simulink model "VCU_CS75_12_16_Test"  (R2014a)
settings: Solver=FixedStepDiscrete  StartTime=0.0  StopTime=25  FixedStep=0.0005  RelTol=1e-3
undefined symbols (not defined in the file): ecucoder_acal, I_SW01_L, LaterlAngleCommand, LDW, RemoteAcclPosition
libraries: simulink x913, ec5744lib x39
(part 17 of 30)

== system VCU_CS75_12_16_Test/长安CS75底盘程序，20ms一次/Output/Subsystem/28A/APA_28A/APA_IncreasePressureReq ==
  APA_IncreasePressureReq : Inport
  APA_IncreasePressureReqRon : Rounding  Operator=round
  APA_IncreasePressureReq_1sat : Saturate  UpperLimit=128  LowerLimit=0
  APA_IncreasePressureReq_Convert : DataTypeConversion  OutDataTypeStr=uint8
  APA_IncreasePressureReq_Convert1 : DataTypeConversion  OutDataTypeStr=uint32
  APA_IncreasePressureReq_D : Product  Inputs=*/
  APA_IncreasePressureReq_F : Constant  OutDataTypeStr=single
  APA_IncreasePressureReq_L : simulink/Logic and Bit Operations/Bitwise Operator  logicop=AND  UseBitMask=on  BitMask=128  BitMaskRealWorld=Stored Integer
  APA_IncreasePressureReq_O : Constant  Value=0  OutDataTypeStr=single
  APA_IncreasePressureReq_S : ArithShift  BitShiftNumber=-7
  APA_IncreasePressureReq_sat : Saturate  UpperLimit=0  LowerLimit=0
  APA_IncreasePressureReq_st : Sum  Inputs=+-
  Constant{1,3..8} (7 alike) : Constant  Value=0  OutDataTypeStr=uint8
  output1 : Outport
  output2 : Outport  Port=2
  output3 : Outport  Port=3
  output4 : Outport  Port=4
  output5 : Outport  Port=5
  output6 : Outport  Port=6
  output7 : Outport  Port=7
  output8 : Outport  Port=8
  wires:
  Constant8/1 -> output8/1
  Constant7/1 -> output7/1
  Constant6/1 -> output6/1
  Constant5/1 -> output5/1
  Constant4/1 -> output4/1
  Constant3/1 -> output3/1
  Constant1/1 -> output1/1
  APA_IncreasePressureReq_Convert/1 -> output2/1
  APA_IncreasePressureReq_L/1 -> APA_IncreasePressureReq_Convert/1
  APA_IncreasePressureReq_Convert1/1 -> APA_IncreasePressureReq_L/1
  APA_IncreasePressureReq_1sat/1 -> APA_IncreasePressureReq_Convert1/1
  APA_IncreasePressureReq_S/1 -> APA_IncreasePressureReq_1sat/1
  APA_IncreasePressureReqRon/1 -> APA_IncreasePressureReq_S/1
  APA_IncreasePressureReq_D/1 -> APA_IncreasePressureReqRon/1
  APA_IncreasePressureReq_F/1 -> APA_IncreasePressureReq_D/2
  APA_IncreasePressureReq_st/1 -> APA_IncreasePressureReq_D/1
  APA_IncreasePressureReq_O/1 -> APA_IncreasePressureReq_st/2
  APA_IncreasePressureReq_sat/1 -> APA_IncreasePressureReq_st/1
  APA_IncreasePressureReq/1 -> APA_IncreasePressureReq_sat/1

== system VCU_CS75_12_16_Test/长安CS75底盘程序，20ms一次/Output/Subsystem/28A/APA_28A/APA_Indication ==
  APA_Indication : Inport
  APA_IndicationRon : Rounding  Operator=round
  APA_Indication_1sat : Saturate  UpperLimit=56  LowerLimit=0
  APA_Indication_Convert : DataTypeConversion  OutDataTypeStr=uint8
  APA_Indication_Convert1 : DataTypeConversion  OutDataTypeStr=uint32
  APA_Indication_D : Product  Inputs=*/
  APA_Indication_F : Constant  OutDataTypeStr=single
  APA_Indication_L : simulink/Logic and Bit Operations/Bitwise Operator  logicop=AND  UseBitMask=on  BitMask=56  BitMaskRealWorld=Stored Integer
  APA_Indication_O : Constant  Value=0  OutDataTypeStr=single
  APA_Indication_S : ArithShift  BitShiftNumber=-3
  APA_Indication_sat : Saturate  UpperLimit=7  LowerLimit=0
  APA_Indication_st : Sum  Inputs=+-
  Constant{2..8} (7 alike) : Constant  Value=0  OutDataTypeStr=uint8
  output1 : Outport
  output2 : Outport  Port=2
  output3 : Outport  Port=3
  output4 : Outport  Port=4
  output5 : Outport  Port=5
  output6 : Outport  Port=6
  output7 : Outport  Port=7
  output8 : Outport  Port=8
  wires:
  Constant8/1 -> output8/1
  Constant7/1 -> output7/1
  Constant6/1 -> output6/1
  Constant5/1 -> output5/1
  Constant4/1 -> output4/1
  Constant3/1 -> output3/1
  Constant2/1 -> output2/1
  APA_Indication_Convert/1 -> output1/1
  APA_Indication_L/1 -> APA_Indication_Convert/1
  APA_Indication_Convert1/1 -> APA_Indication_L/1
  APA_Indication_1sat/1 -> APA_Indication_Convert1/1
  APA_Indication_S/1 -> APA_Indication_1sat/1
  APA_IndicationRon/1 -> APA_Indication_S/1
  APA_Indication_D/1 -> APA_IndicationRon/1
  APA_Indication_F/1 -> APA_Indication_D/2
  APA_Indication_st/1 -> APA_Indication_D/1
  APA_Indication_O/1 -> APA_Indication_st/2
  APA_Indication_sat/1 -> APA_Indication_st/1
  APA_Indication/1 -> APA_Indication_sat/1

== system VCU_CS75_12_16_Test/长安CS75底盘程序，20ms一次/Output/Subsystem/28A/APA_28A/APA_OnOff ==
  APA_OnOff : Inport
  APA_OnOffRon : Rounding  Operator=round
  APA_OnOff_1sat : Saturate  UpperLimit=64  LowerLimit=0
  APA_OnOff_Convert : DataTypeConversion  OutDataTypeStr=uint8
  APA_OnOff_Convert1 : DataTypeConversion  OutDataTypeStr=uint32
  APA_OnOff_D : Product  Inputs=*/
  APA_OnOff_F : Constant  OutDataTypeStr=single
  APA_OnOff_L : simulink/Logic and Bit Operations/Bitwise Operator  logicop=AND  UseBitMask=on  BitMask=64  BitMaskRealWorld=Stored Integer
  APA_OnOff_O : Constant  Value=0  OutDataTypeStr=single
  APA_OnOff_S : ArithShift  BitShiftNumber=-6
  APA_OnOff_sat : Saturate  UpperLimit=0  LowerLimit=0
  APA_OnOff_st : Sum  Inputs=+-
  Constant{2..8} (7 alike) : Constant  Value=0  OutDataTypeStr=uint8
  output1 : Outport
  output2 : Outport  Port=2
  output3 : Outport  Port=3
  output4 : Outport  Port=4
  output5 : Outport  Port=5
  output6 : Outport  Port=6
  output7 : Outport  Port=7
  output8 : Outport  Port=8
  wires:
  Constant8/1 -> output8/1
  Constant7/1 -> output7/1
  Constant6/1 -> output6/1
  Constant5/1 -> output5/1
  Constant4/1 -> output4/1
  Constant3/1 -> output3/1
  Constant2/1 -> output2/1
  APA_OnOff_Convert/1 -> output1/1
  APA_OnOff_L/1 -> APA_OnOff_Convert/1
  APA_OnOff_Convert1/1 -> APA_OnOff_L/1
  APA_OnOff_1sat/1 -> APA_OnOff_Convert1/1
  APA_OnOff_S/1 -> APA_OnOff_1sat/1
  APA_OnOffRon/1 -> APA_OnOff_S/1
  APA_OnOff_D/1 -> APA_OnOffRon/1
  APA_OnOff_F/1 -> APA_OnOff_D/2
  APA_OnOff_st/1 -> APA_OnOff_D/1
  APA_OnOff_O/1 -> APA_OnOff_st/2
  APA_OnOff_sat/1 -> APA_OnOff_st/1
  APA_OnOff/1 -> APA_OnOff_sat/1

== system VCU_CS75_12_16_Test/长安CS75底盘程序，20ms一次/Output/Subsystem/28A/APA_28A/APA_RollingCounter ==
  APA_RollingCounter : Inport
  APA_RollingCounterRon : Rounding  Operator=round
  APA_RollingCounter_1sat : Saturate  UpperLimit=15  LowerLimit=0
  APA_RollingCounter_Convert : DataTypeConversion  OutDataTypeStr=uint8
  APA_RollingCounter_Convert1 : DataTypeConversion  OutDataTypeStr=uint32
  APA_RollingCounter_D : Product  Inputs=*/
  APA_RollingCounter_F : Constant  OutDataTypeStr=single
  APA_RollingCounter_L : simulink/Logic and Bit Operations/Bitwise Operator  logicop=AND  UseBitMask=on  BitMask=15  BitMaskRealWorld=Stored Integer
  APA_RollingCounter_O : Constant  Value=0  OutDataTypeStr=single
  APA_RollingCounter_S : ArithShift
  APA_RollingCounter_sat : Saturate  UpperLimit=15  LowerLimit=0
  APA_RollingCounter_st : Sum  Inputs=+-
  Constant{1..6,8} (7 alike) : Constant  Value=0  OutDataTypeStr=uint8
  output1 : Outport
  output2 : Outport  Port=2
  output3 : Outport  Port=3
  output4 : Outport  Port=4
  output5 : Outport  Port=5
  output6 : Outport  Port=6
  output7 : Outport  Port=7
  output8 : Outport  Port=8
  wires:
  Constant8/1 -> output8/1
  Constant6/1 -> output6/1
  Constant5/1 -> output5/1
  Constant4/1 -> output4/1
  Constant3/1 -> output3/1
  Constant2/1 -> output2/1
  Constant1/1 -> output1/1
  APA_RollingCounter_Convert/1 -> output7/1
  APA_RollingCounter_L/1 -> APA_RollingCounter_Convert/1
  APA_RollingCounter_Convert1/1 -> APA_RollingCounter_L/1
  APA_RollingCounter_1sat/1 -> APA_RollingCounter_Convert1/1
  APA_RollingCounter_S/1 -> APA_RollingCounter_1sat/1
  APA_RollingCounterRon/1 -> APA_RollingCounter_S/1
  APA_RollingCounter_D/1 -> APA_RollingCounterRon/1
  APA_RollingCounter_F/1 -> APA_RollingCounter_D/2
  APA_RollingCounter_st/1 -> APA_RollingCounter_D/1
  APA_RollingCounter_O/1 -> APA_RollingCounter_st/2
  APA_RollingCounter_sat/1 -> APA_RollingCounter_st/1
  APA_RollingCounter/1 -> APA_RollingCounter_sat/1

== system VCU_CS75_12_16_Test/长安CS75底盘程序，20ms一次/Output/Subsystem/28A/APA_28A/APA_SteeringAngleReqProtection ==
  APA_SteeringAngleReqProtection : Inport
  APA_SteeringAngleReqProtectionRon : Rounding  Operator=round
  APA_SteeringAngleReqProtection_1sat : Saturate  UpperLimit=3  LowerLimit=0
  APA_SteeringAngleReqProtection_Convert : DataTypeConversion  OutDataTypeStr=uint8
  APA_SteeringAngleReqProtection_Convert1 : DataTypeConversion  OutDataTypeStr=uint32
  APA_SteeringAngleReqProtection_D : Product  Inputs=*/
  APA_SteeringAngleReqProtection_F : Constant  OutDataTypeStr=single
  APA_SteeringAngleReqProtection_L : simulink/Logic and Bit Operations/Bitwise Operator  logicop=AND  UseBitMask=on  BitMask=3  BitMaskRealWorld=Stored Integer
  APA_SteeringAngleReqProtection_O : Constant  Value=0  OutDataTypeStr=single
  APA_SteeringAngleReqProtection_S : ArithShift
  APA_SteeringAngleReqProtection_sat : Saturate  UpperLimit=3  LowerLimit=0
  APA_SteeringAngleReqProtection_st : Sum  Inputs=+-
  Constant{1..4,6..8} (7 alike) : Constant  Value=0  OutDataTypeStr=uint8
  output1 : Outport
  output2 : Outport  Port=2
  output3 : Outport  Port=3
  output4 : Outport  Port=4
  output5 : Outport  Port=5
  output6 : Outport  Port=6
  output7 : Outport  Port=7
  output8 : Outport  Port=8
  wires:
  Constant8/1 -> output8/1
  Constant7/1 -> output7/1
  Constant6/1 -> output6/1
  Constant4/1 -> output4/1
  Constant3/1 -> output3/1
  Constant2/1 -> output2/1
  Constant1/1 -> output1/1
  APA_SteeringAngleReqProtection_Convert/1 -> output5/1
  APA_SteeringAngleReqProtection_L/1 -> APA_SteeringAngleReqProtection_Convert/1
  APA_SteeringAngleReqProtection_Convert1/1 -> APA_SteeringAngleReqProtection_L/1
  APA_SteeringAngleReqProtection_1sat/1 -> APA_SteeringAngleReqProtection_Convert1/1
  APA_SteeringAngleReqProtection_S/1 -> APA_SteeringAngleReqProtection_1sat/1
  APA_SteeringAngleReqProtectionRon/1 -> APA_SteeringAngleReqProtection_S/1
  APA_SteeringAngleReqProtection_D/1 -> APA_SteeringAngleReqProtectionRon/1
  APA_SteeringAngleReqProtection_F/1 -> APA_SteeringAngleReqProtection_D/2
  APA_SteeringAngleReqProtection_st/1 -> APA_SteeringAngleReqProtection_D/1
  APA_SteeringAngleReqProtection_O/1 -> APA_SteeringAngleReqProtection_st/2
  APA_SteeringAngleReqProtection_sat/1 -> APA_SteeringAngleReqProtection_st/1
  APA_SteeringAngleReqProtection/1 -> APA_SteeringAngleReqProtection_sat/1

== system VCU_CS75_12_16_Test/长安CS75底盘程序，20ms一次/Output/Subsystem/28D/LAS_28D/CRC ==
  CRC : Inport
  CRCRon : Rounding  Operator=round
  CRC_1sat : Saturate  UpperLimit=255  LowerLimit=0
  CRC_Convert : DataTypeConversion  OutDataTypeStr=uint8
  CRC_Convert1 : DataTypeConversion  OutDataTypeStr=uint32
  CRC_D : Product  Inputs=*/
  CRC_F : Constant  OutDataTypeStr=single
  CRC_L : simulink/Logic and Bit Operations/Bitwise Operator  logicop=AND  UseBitMask=on  BitMask=255  BitMaskRealWorld=Stored Integer
  CRC_O : Constant  Value=0  OutDataTypeStr=single
  CRC_S : ArithShift
  CRC_sat : Saturate  UpperLimit=0  LowerLimit=0
  CRC_st : Sum  Inputs=+-
  Constant{1..7} (7 alike) : Constant  Value=0  OutDataTypeStr=uint8
  output1 : Outport
  output2 : Outport  Port=2
  output3 : Outport  Port=3
  output4 : Outport  Port=4
  output5 : Outport  Port=5
  output6 : Outport  Port=6
  output7 : Outport  Port=7
  output8 : Outport  Port=8
  wires:
  CRC/1 -> CRC_sat/1
  CRC_sat/1 -> CRC_st/1
  CRC_O/1 -> CRC_st/2
  CRC_st/1 -> CRC_D/1
  CRC_F/1 -> CRC_D/2
  CRC_D/1 -> CRCRon/1
  CRCRon/1 -> CRC_S/1
  CRC_S/1 -> CRC_1sat/1
  CRC_1sat/1 -> CRC_Convert1/1
  CRC_Convert1/1 -> CRC_L/1
  CRC_L/1 -> CRC_Convert/1
  CRC_Convert/1 -> output8/1
  Constant1/1 -> output1/1
  Constant2/1 -> output2/1
  Constant3/1 -> output3/1
  Constant4/1 -> output4/1
  Constant5/1 -> output5/1
  Constant6/1 -> output6/1
  Constant7/1 -> output7/1

== system VCU_CS75_12_16_Test/长安CS75底盘程序，20ms一次/Output/Subsystem/28D/LAS_28D/LAS_CaliStatus ==
  LAS_CaliStatus : Inport
  Constant{1,3..8} (7 alike) : Constant  Value=0  OutDataTypeStr=uint8
  LAS_CaliStatusRon : Rounding  Operator=round
  LAS_CaliStatus_1sat : Saturate  UpperLimit=3  LowerLimit=0
  LAS_CaliStatus_Convert : DataTypeConversion  OutDataTypeStr=uint8
  LAS_CaliStatus_Convert1 : DataTypeConversion  OutDataTypeStr=uint32
  LAS_CaliStatus_D : Product  Inputs=*/
  LAS_CaliStatus_F : Constant  OutDataTypeStr=single
  LAS_CaliStatus_L : simulink/Logic and Bit Operations/Bitwise Operator  logicop=AND  UseBitMask=on  BitMask=3  BitMaskRealWorld=Stored Integer
  LAS_CaliStatus_O : Constant  Value=0  OutDataTypeStr=single
  LAS_CaliStatus_S : ArithShift
  LAS_CaliStatus_sat : Saturate  UpperLimit=0  LowerLimit=0
  LAS_CaliStatus_st : Sum  Inputs=+-
  output1 : Outport
  output2 : Outport  Port=2
  output3 : Outport  Port=3
  output4 : Outport  Port=4
  output5 : Outport  Port=5
  output6 : Outport  Port=6
  output7 : Outport  Port=7
  output8 : Outport  Port=8
  wires:
  LAS_CaliStatus/1 -> LAS_CaliStatus_sat/1
  LAS_CaliStatus_sat/1 -> LAS_CaliStatus_st/1
  LAS_CaliStatus_O/1 -> LAS_CaliStatus_st/2
  LAS_CaliStatus_st/1 -> LAS_CaliStatus_D/1
  LAS_CaliStatus_F/1 -> LAS_CaliStatus_D/2
  LAS_CaliStatus_D/1 -> LAS_CaliStatusRon/1
  LAS_CaliStatusRon/1 -> LAS_CaliStatus_S/1
  LAS_CaliStatus_S/1 -> LAS_CaliStatus_1sat/1
  LAS_CaliStatus_1sat/1 -> LAS_CaliStatus_Convert1/1
  LAS_CaliStatus_Convert1/1 -> LAS_CaliStatus_L/1
  LAS_CaliStatus_L/1 -> LAS_CaliStatus_Convert/1
  LAS_CaliStatus_Convert/1 -> output2/1
  Constant1/1 -> output1/1
  Constant3/1 -> output3/1
  Constant4/1 -> output4/1
  Constant5/1 -> output5/1
  Constant6/1 -> output6/1
  Constant7/1 -> output7/1
  Constant8/1 -> output8/1

== system VCU_CS75_12_16_Test/长安CS75底盘程序，20ms一次/Output/Subsystem/28D/LAS_28D/LAS_DFDFailed ==
  LAS_DFDFailed : Inport
  Constant{1,3..8} (7 alike) : Constant  Value=0  OutDataTypeStr=uint8
  LAS_DFDFailedRon : Rounding  Operator=round
  LAS_DFDFailed_1sat : Saturate  UpperLimit=8  LowerLimit=0
  LAS_DFDFailed_Convert : DataTypeConversion  OutDataTypeStr=uint8
  LAS_DFDFailed_Convert1 : DataTypeConversion  OutDataTypeStr=uint32
  LAS_DFDFailed_D : Product  Inputs=*/
  LAS_DFDFailed_F : Constant  OutDataTypeStr=single
  LAS_DFDFailed_L : simulink/Logic and Bit Operations/Bitwise Operator  logicop=AND  UseBitMask=on  BitMask=8  BitMaskRealWorld=Stored Integer
  LAS_DFDFailed_O : Constant  Value=0  OutDataTypeStr=single
  LAS_DFDFailed_S : ArithShift  BitShiftNumber=-3
  LAS_DFDFailed_sat : Saturate  UpperLimit=0  LowerLimit=0
  LAS_DFDFailed_st : Sum  Inputs=+-
  output1 : Outport
  output2 : Outport  Port=2
  output3 : Outport  Port=3
  output4 : Outport  Port=4
  output5 : Outport  Port=5
  output6 : Outport  Port=6
  output7 : Outport  Port=7
  output8 : Outport  Port=8
  wires:
  LAS_DFDFailed/1 -> LAS_DFDFailed_sat/1
  LAS_DFDFailed_sat/1 -> LAS_DFDFailed_st/1
  LAS_DFDFailed_O/1 -> LAS_DFDFailed_st/2
  LAS_DFDFailed_st/1 -> LAS_DFDFailed_D/1
  LAS_DFDFailed_F/1 -> LAS_DFDFailed_D/2
  LAS_DFDFailed_D/1 -> LAS_DFDFailedRon/1
  LAS_DFDFailedRon/1 -> LAS_DFDFailed_S/1
  LAS_DFDFailed_S/1 -> LAS_DFDFailed_1sat/1
  LAS_DFDFailed_1sat/1 -> LAS_DFDFailed_Convert1/1
  LAS_DFDFailed_Convert1/1 -> LAS_DFDFailed_L/1
  LAS_DFDFailed_L/1 -> LAS_DFDFailed_Convert/1
  LAS_DFDFailed_Convert/1 -> output2/1
  Constant1/1 -> output1/1
  Constant3/1 -> output3/1
  Constant4/1 -> output4/1
  Constant5/1 -> output5/1
  Constant6/1 -> output6/1
  Constant7/1 -> output7/1
  Constant8/1 -> output8/1

== system VCU_CS75_12_16_Test/长安CS75底盘程序，20ms一次/Output/Subsystem/28D/LAS_28D/LAS_DFDWarning ==
  LAS_DFDWarning : Inport
  Constant{1..3,5..8} (7 alike) : Constant  Value=0  OutDataTypeStr=uint8
  LAS_DFDWarningRon : Rounding  Operator=round
  LAS_DFDWarning_1sat : Saturate  UpperLimit=3  LowerLimit=0
  LAS_DFDWarning_Convert : DataTypeConversion  OutDataTypeStr=uint8
  LAS_DFDWarning_Convert1 : DataTypeConversion  OutDataTypeStr=uint32
  LAS_DFDWarning_D : Product  Inputs=*/
  LAS_DFDWarning_F : Constant  OutDataTypeStr=single
  LAS_DFDWarning_L : simulink/Logic and Bit Operations/Bitwise Operator  logicop=AND  UseBitMask=on  BitMask=3  BitMaskRealWorld=Stored Integer
  LAS_DFDWarning_O : Constant  Value=0  OutDataTypeStr=single
  LAS_DFDWarning_S : ArithShift
  LAS_DFDWarning_sat : Saturate  UpperLimit=0  LowerLimit=0
  LAS_DFDWarning_st : Sum  Inputs=+-
  output1 : Outport
  output2 : Outport  Port=2
  output3 : Outport  Port=3
  output4 : Outport  Port=4
  output5 : Outport  Port=5
  output6 : Outport  Port=6
  output7 : Outport  Port=7
  output8 : Outport  Port=8
  wires:
  LAS_DFDWarning/1 -> LAS_DFDWarning_sat/1
  LAS_DFDWarning_sat/1 -> LAS_DFDWarning_st/1
  LAS_DFDWarning_O/1 -> LAS_DFDWarning_st/2
  LAS_DFDWarning_st/1 -> LAS_DFDWarning_D/1
  LAS_DFDWarning_F/1 -> LAS_DFDWarning_D/2
  LAS_DFDWarning_D/1 -> LAS_DFDWarningRon/1
  LAS_DFDWarningRon/1 -> LAS_DFDWarning_S/1
  LAS_DFDWarning_S/1 -> LAS_DFDWarning_1sat/1
  LAS_DFDWarning_1sat/1 -> LAS_DFDWarning_Convert1/1
  LAS_DFDWarning_Convert1/1 -> LAS_DFDWarning_L/1
  LAS_DFDWarning_L/1 -> LAS_DFDWarning_Convert/1
  LAS_DFDWarning_Convert/1 -> output4/1
  Constant1/1 -> output1/1
  Constant2/1 -> output2/1
  Constant3/1 -> output3/1
  Constant5/1 -> output5/1
  Constant6/1 -> output6/1
  Constant7/1 -> output7/1
  Constant8/1 -> output8/1

== system VCU_CS75_12_16_Test/长安CS75底盘程序，20ms一次/Output/Subsystem/28D/LAS_28D/LAS_LASFailed ==
  LAS_LASFailed : Inport
  Constant{1..3,5..8} (7 alike) : Constant  Value=0  OutDataTypeStr=uint8
  LAS_LASFailedRon : Rounding  Operator=round
  LAS_LASFailed_1sat : Saturate  UpperLimit=12  LowerLimit=0
  LAS_LASFailed_Convert : DataTypeConversion  OutDataTypeStr=uint8
  LAS_LASFailed_Convert1 : DataTypeConversion  OutDataTypeStr=uint32
  LAS_LASFailed_D : Product  Inputs=*/
  LAS_LASFailed_F : Constant  OutDataTypeStr=single
  LAS_LASFailed_L : simulink/Logic and Bit Operations/Bitwise Operator  logicop=AND  UseBitMask=on  BitMask=12  BitMaskRealWorld=Stored Integer
  LAS_LASFailed_O : Constant  Value=0  OutDataTypeStr=single
  LAS_LASFailed_S : ArithShift  BitShiftNumber=-2
  LAS_LASFailed_sat : Saturate  UpperLimit=0  LowerLimit=0
  LAS_LASFailed_st : Sum  Inputs=+-
  output1 : Outport
  output2 : Outport  Port=2
  output3 : Outport  Port=3
  output4 : Outport  Port=4
  output5 : Outport  Port=5
  output6 : Outport  Port=6
  output7 : Outport  Port=7
  output8 : Outport  Port=8
  wires:
  LAS_LASFailed/1 -> LAS_LASFailed_sat/1
  LAS_LASFailed_sat/1 -> LAS_LASFailed_st/1
  LAS_LASFailed_O/1 -> LAS_LASFailed_st/2
  LAS_LASFailed_st/1 -> LAS_LASFailed_D/1
  LAS_LASFailed_F/1 -> LAS_LASFailed_D/2
  LAS_LASFailed_D/1 -> LAS_LASFailedRon/1
  LAS_LASFailedRon/1 -> LAS_LASFailed_S/1
  LAS_LASFailed_S/1 -> LAS_LASFailed_1sat/1
  LAS_LASFailed_1sat/1 -> LAS_LASFailed_Convert1/1
  LAS_LASFailed_Convert1/1 -> LAS_LASFailed_L/1
  LAS_LASFailed_L/1 -> LAS_LASFailed_Convert/1
  LAS_LASFailed_Convert/1 -> output4/1
  Constant1/1 -> output1/1
  Constant2/1 -> output2/1
  Constant3/1 -> output3/1
  Constant5/1 -> output5/1
  Constant6/1 -> output6/1
  Constant7/1 -> output7/1
  Constant8/1 -> output8/1

== system VCU_CS75_12_16_Test/长安CS75底盘程序，20ms一次/Output/Subsystem/28D/LAS_28D/LAS_LDWReminder ==
  LAS_LDWReminder : Inport
  Constant{1..2,4..8} (7 alike) : Constant  Value=0  OutDataTypeStr=uint8
  LAS_LDWReminderRon : Rounding  Operator=round
  LAS_LDWReminder_1sat : Saturate  UpperLimit=96  LowerLimit=0
  LAS_LDWReminder_Convert : DataTypeConversion  OutDataTypeStr=uint8
  LAS_LDWReminder_Convert1 : DataTypeConversion  OutDataTypeStr=uint32
  LAS_LDWReminder_D : Product  Inputs=*/
  LAS_LDWReminder_F : Constant  OutDataTypeStr=single
  LAS_LDWReminder_L : simulink/Logic and Bit Operations/Bitwise Operator  logicop=AND  UseBitMask=on  BitMask=96  BitMaskRealWorld=Stored Integer
  LAS_LDWReminder_O : Constant  Value=0  OutDataTypeStr=single
  LAS_LDWReminder_S : ArithShift  BitShiftNumber=-5
  LAS_LDWReminder_sat : Saturate  UpperLimit=0  LowerLimit=0
  LAS_LDWReminder_st : Sum  Inputs=+-
  output1 : Outport
  output2 : Outport  Port=2
  output3 : Outport  Port=3
  output4 : Outport  Port=4
  output5 : Outport  Port=5
  output6 : Outport  Port=6
  output7 : Outport  Port=7
  output8 : Outport  Port=8
  wires:
  LAS_LDWReminder/1 -> LAS_LDWReminder_sat/1
  LAS_LDWReminder_sat/1 -> LAS_LDWReminder_st/1
  LAS_LDWReminder_O/1 -> LAS_LDWReminder_st/2
  LAS_LDWReminder_st/1 -> LAS_LDWReminder_D/1
  LAS_LDWReminder_F/1 -> LAS_LDWReminder_D/2
  LAS_LDWReminder_D/1 -> LAS_LDWReminderRon/1
  LAS_LDWReminderRon/1 -> LAS_LDWReminder_S/1
  LAS_LDWReminder_S/1 -> LAS_LDWReminder_1sat/1
  LAS_LDWReminder_1sat/1 -> LAS_LDWReminder_Convert1/1
  LAS_LDWReminder_Convert1/1 -> LAS_LDWReminder_L/1
  LAS_LDWReminder_L/1 -> LAS_LDWReminder_Convert/1
  LAS_LDWReminder_Convert/1 -> output3/1
  Constant1/1 -> output1/1
  Constant2/1 -> output2/1
  Constant4/1 -> output4/1
  Constant5/1 -> output5/1
  Constant6/1 -> output6/1
  Constant7/1 -> output7/1
  Constant8/1 -> output8/1

== system VCU_CS75_12_16_Test/长安CS75底盘程序，20ms一次/Output/Subsystem/28D/LAS_28D/LAS_LDWStatus ==
  LAS_LDWStatus : Inport
  Constant{2..8} (7 alike) : Constant  Value=0  OutDataTypeStr=uint8
  LAS_LDWStatusRon : Rounding  Operator=round
  LAS_LDWStatus_1sat : Saturate  UpperLimit=96  LowerLimit=0
  LAS_LDWStatus_Convert : DataTypeConversion  OutDataTypeStr=uint8
  LAS_LDWStatus_Convert1 : DataTypeConversion  OutDataTypeStr=uint32
  LAS_LDWStatus_D : Product  Inputs=*/
  LAS_LDWStatus_F : Constant  OutDataTypeStr=single
  LAS_LDWStatus_L : simulink/Logic and Bit Operations/Bitwise Operator  logicop=AND  UseBitMask=on  BitMask=96  BitMaskRealWorld=Stored Integer
  LAS_LDWStatus_O : Constant  Value=0  OutDataTypeStr=single
  LAS_LDWStatus_S : ArithShift  BitShiftNumber=-5
  LAS_LDWStatus_sat : Saturate  UpperLimit=3  LowerLimit=0
  LAS_LDWStatus_st : Sum  Inputs=+-
  output1 : Outport
  output2 : Outport  Port=2
  output3 : Outport  Port=3
  output4 : Outport  Port=4
  output5 : Outport  Port=5
  output6 : Outport  Port=6
  output7 : Outport  Port=7
  output8 : Outport  Port=8
  wires:
  LAS_LDWStatus/1 -> LAS_LDWStatus_sat/1
  LAS_LDWStatus_sat/1 -> LAS_LDWStatus_st/1
  LAS_LDWStatus_O/1 -> LAS_LDWStatus_st/2
  LAS_LDWStatus_st/1 -> LAS_LDWStatus_D/1
  LAS_LDWStatus_F/1 -> LAS_LDWStatus_D/2
  LAS_LDWStatus_D/1 -> LAS_LDWStatusRon/1
  LAS_LDWStatusRon/1 -> LAS_LDWStatus_S/1
  LAS_LDWStatus_S/1 -> LAS_LDWStatus_1sat/1
  LAS_LDWStatus_1sat/1 -> LAS_LDWStatus_Convert1/1
  LAS_LDWStatus_Convert1/1 -> LAS_LDWStatus_L/1
  LAS_LDWStatus_L/1 -> LAS_LDWStatus_Convert/1
  LAS_LDWStatus_Convert/1 -> output1/1
  Constant2/1 -> output2/1
  Constant3/1 -> output3/1
  Constant4/1 -> output4/1
  Constant5/1 -> output5/1
  Constant6/1 -> output6/1
  Constant7/1 -> output7/1
  Constant8/1 -> output8/1

== system VCU_CS75_12_16_Test/长安CS75底盘程序，20ms一次/Output/Subsystem/28D/LAS_28D/LAS_LDWVibrationWarning ==
  LAS_LDWVibrationWarning : Inport
  Constant{1,3..8} (7 alike) : Constant  Value=0  OutDataTypeStr=uint8
  LAS_LDWVibrationWarningRon : Rounding  Operator=round
  LAS_LDWVibrationWarning_1sat : Saturate  UpperLimit=96  LowerLimit=0
  LAS_LDWVibrationWarning_Convert : DataTypeConversion  OutDataTypeStr=uint8
  LAS_LDWVibrationWarning_Convert1 : DataTypeConversion  OutDataTypeStr=uint32
  LAS_LDWVibrationWarning_D : Product  Inputs=*/
  LAS_LDWVibrationWarning_F : Constant  OutDataTypeStr=single
  LAS_LDWVibrationWarning_L : simulink/Logic and Bit Operations/Bitwise Operator  logicop=AND  UseBitMask=on  BitMask=96  BitMaskRealWorld=Stored Integer
  LAS_LDWVibrationWarning_O : Constant  Value=0  OutDataTypeStr=single
  LAS_LDWVibrationWarning_S : ArithShift  BitShiftNumber=-5
  LAS_LDWVibrationWarning_sat : Saturate  UpperLimit=0  LowerLimit=0
  LAS_LDWVibrationWarning_st : Sum  Inputs=+-
  output1 : Outport
  output2 : Outport  Port=2
  output3 : Outport  Port=3
  output4 : Outport  Port=4
  output5 : Outport  Port=5
  output6 : Outport  Port=6
  output7 : Outport  Port=7
  output8 : Outport  Port=8
  wires:
  LAS_LDWVibrationWarning/1 -> LAS_LDWVibrationWarning_sat/1
  LAS_LDWVibrationWarning_sat/1 -> LAS_LDWVibrationWarning_st/1
  LAS_LDWVibrationWarning_O/1 -> LAS_LDWVibrationWarning_st/2
  LAS_LDWVibrationWarning_st/1 -> LAS_LDWVibrationWarning_D/1
  LAS_LDWVibrationWarning_F/1 -> LAS_LDWVibrationWarning_D/2
  LAS_LDWVibrationWarning_D/1 -> LAS_LDWVibrationWarningRon/1
  LAS_LDWVibrationWarningRon/1 -> LAS_LDWVibrationWarning_S/1
  LAS_LDWVibrationWarning_S/1 -> LAS_LDWVibrationWarning_1sat/1
  LAS_LDWVibrationWarning_1sat/1 -> LAS_LDWVibrationWarning_Convert1/1
  LAS_LDWVibrationWarning_Convert1/1 -> LAS_LDWVibrationWarning_L/1
  LAS_LDWVibrationWarning_L/1 -> LAS_LDWVibrationWarning_Convert/1
  LAS_LDWVibrationWarning_Convert/1 -> output2/1
  Constant1/1 -> output1/1
  Constant3/1 -> output3/1
  Constant4/1 -> output4/1
  Constant5/1 -> output5/1
  Constant6/1 -> output6/1
  Constant7/1 -> output7/1
  Constant8/1 -> output8/1

== system VCU_CS75_12_16_Test/长安CS75底盘程序，20ms一次/Output/Subsystem/28D/LAS_28D/LAS_LKSStatus ==
  LAS_LKSStatus : Inport
  Constant{1..4,6..8} (7 alike) : Constant  Value=0  OutDataTypeStr=uint8
  LAS_LKSStatusRon : Rounding  Operator=round
  LAS_LKSStatus_1sat : Saturate  UpperLimit=224  LowerLimit=0
  LAS_LKSStatus_Convert : DataTypeConversion  OutDataTypeStr=uint8
  LAS_LKSStatus_Convert1 : DataTypeConversion  OutDataTypeStr=uint32
  LAS_LKSStatus_D : Product  Inputs=*/
  LAS_LKSStatus_F : Constant  OutDataTypeStr=single
  LAS_LKSStatus_L : simulink/Logic and Bit Operations/Bitwise Operator  logicop=AND  UseBitMask=on  BitMask=224  BitMaskRealWorld=Stored Integer
  LAS_LKSStatus_O : Constant  Value=0  OutDataTypeStr=single
  LAS_LKSStatus_S : ArithShift  BitShiftNumber=-5
  LAS_LKSStatus_sat : Saturate  UpperLimit=0  LowerLimit=0
  LAS_LKSStatus_st : Sum  Inputs=+-
  output1 : Outport
  output2 : Outport  Port=2
  output3 : Outport  Port=3
  output4 : Outport  Port=4
  output5 : Outport  Port=5
  output6 : Outport  Port=6
  output7 : Outport  Port=7
  output8 : Outport  Port=8
  wires:
  LAS_LKSStatus/1 -> LAS_LKSStatus_sat/1
  LAS_LKSStatus_sat/1 -> LAS_LKSStatus_st/1
  LAS_LKSStatus_O/1 -> LAS_LKSStatus_st/2
  LAS_LKSStatus_st/1 -> LAS_LKSStatus_D/1
  LAS_LKSStatus_F/1 -> LAS_LKSStatus_D/2
  LAS_LKSStatus_D/1 -> LAS_LKSStatusRon/1
  LAS_LKSStatusRon/1 -> LAS_LKSStatus_S/1
  LAS_LKSStatus_S/1 -> LAS_LKSStatus_1sat/1
  LAS_LKSStatus_1sat/1 -> LAS_LKSStatus_Convert1/1
  LAS_LKSStatus_Convert1/1 -> LAS_LKSStatus_L/1
  LAS_LKSStatus_L/1 -> LAS_LKSStatus_Convert/1
  LAS_LKSStatus_Convert/1 -> output5/1
  Constant1/1 -> output1/1
  Constant2/1 -> output2/1
  Constant3/1 -> output3/1
  Constant4/1 -> output4/1
  Constant6/1 -> output6/1
  Constant7/1 -> output7/1
  Constant8/1 -> output8/1

== system VCU_CS75_12_16_Test/长安CS75底盘程序，20ms一次/Output/Subsystem/28D/LAS_28D/LAS_SLASpdLimit ==
  LAS_SLASpdLimit : Inport
  Constant{1..2,5..8} (6 alike) : Constant  Value=0  OutDataTypeStr=uint8
  LAS_SLASpdLimitBitCov : DataTypeConversion  OutDataTypeStr=uint8
  LAS_SLASpdLimitCOV : DataTypeConversion  OutDataTypeStr=uint8
  LAS_SLASpdLimitRon : Rounding  Operator=round
  LAS_SLASpdLimit_1sat : Saturate  UpperLimit=4080  LowerLimit=0
  LAS_SLASpdLimit_And : simulink/Logic and Bit Operations/Bitwise Operator  logicop=AND  UseBitMask=off  NumInputPorts=2  BitMask=bin2dec('11011001')  BitMaskRealWorld=Stored Integer
  LAS_SLASpdLimit_And_C : Constant  Value=255  OutDataTypeStr=uint32
  LAS_SLASpdLimit_Convert : DataTypeConversion  OutDataTypeStr=uint32
  LAS_SLASpdLimit_D : Product  Inputs=*/
  LAS_SLASpdLimit_D1 : Product  Inputs=*/
  LAS_SLASpdLimit_F : Constant  OutDataTypeStr=single
  LAS_SLASpdLimit_L : simulink/Logic and Bit Operations/Bitwise Operator  logicop=AND  UseBitMask=on  BitMask=4080  BitMaskRealWorld=Stored Integer
  LAS_SLASpdLimit_O : Constant  Value=0  OutDataTypeStr=single
  LAS_SLASpdLimit_S : ArithShift  BitShiftNumber=-4
  LAS_SLASpdLimit_sat : Saturate  UpperLimit=0  LowerLimit=0
  LAS_SLASpdLimit_st : Sum  Inputs=+-
  LAS_SLASpdLimitoutput3_C : Constant  Value=256
  output1 : Outport
  output2 : Outport  Port=2
  output3 : Outport  Port=3
  output4 : Outport  Port=4
  output5 : Outport  Port=5
  output6 : Outport  Port=6
  output7 : Outport  Port=7
  output8 : Outport  Port=8
  wires:
  LAS_SLASpdLimit/1 -> LAS_SLASpdLimit_sat/1
  LAS_SLASpdLimit_sat/1 -> LAS_SLASpdLimit_st/1
  LAS_SLASpdLimit_O/1 -> LAS_SLASpdLimit_st/2
  LAS_SLASpdLimit_st/1 -> LAS_SLASpdLimit_D/1
  LAS_SLASpdLimit_F/1 -> LAS_SLASpdLimit_D/2
  LAS_SLASpdLimit_D/1 -> LAS_SLASpdLimitRon/1
  LAS_SLASpdLimitRon/1 -> LAS_SLASpdLimit_S/1
  LAS_SLASpdLimit_S/1 -> LAS_SLASpdLimit_1sat/1
  LAS_SLASpdLimit_1sat/1 -> LAS_SLASpdLimit_Convert/1
  LAS_SLASpdLimit_Convert/1 -> LAS_SLASpdLimit_L/1
  LAS_SLASpdLimit_L/1 -> LAS_SLASpdLimit_D1/1, LAS_SLASpdLimit_And/1
  LAS_SLASpdLimitoutput3_C/1 -> LAS_SLASpdLimit_D1/2
  LAS_SLASpdLimit_D1/1 -> LAS_SLASpdLimitCOV/1
  LAS_SLASpdLimitCOV/1 -> output3/1
  LAS_SLASpdLimit_And_C/1 -> LAS_SLASpdLimit_And/2
  LAS_SLASpdLimit_And/1 -> LAS_SLASpdLimitBitCov/1
  LAS_SLASpdLimitBitCov/1 -> output4/1
  Constant1/1 -> output1/1
  Constant2/1 -> output2/1
  Constant5/1 -> output5/1
  Constant6/1 -> output6/1
  Constant7/1 -> output7/1
  Constant8/1 -> output8/1

== system VCU_CS75_12_16_Test/长安CS75底盘程序，20ms一次/Output/Subsystem/28D/LAS_28D/LAS_SLASpdLimitUnit ==
  LAS_SLASpdLimitUnit : Inport
  Constant{2..8} (7 alike) : Constant  Value=0  OutDataTypeStr=uint8
  LAS_SLASpdLimitUnitRon : Rounding  Operator=round
  LAS_SLASpdLimitUnit_1sat : Saturate  UpperLimit=12  LowerLimit=0
  LAS_SLASpdLimitUnit_Convert : DataTypeConversion  OutDataTypeStr=uint8
  LAS_SLASpdLimitUnit_Convert1 : DataTypeConversion  OutDataTypeStr=uint32
  LAS_SLASpdLimitUnit_D : Product  Inputs=*/
  LAS_SLASpdLimitUnit_F : Constant  OutDataTypeStr=single
  LAS_SLASpdLimitUnit_L : simulink/Logic and Bit Operations/Bitwise Operator  logicop=AND  UseBitMask=on  BitMask=12  BitMaskRealWorld=Stored Integer
  LAS_SLASpdLimitUnit_O : Constant  Value=0  OutDataTypeStr=single
  LAS_SLASpdLimitUnit_S : ArithShift  BitShiftNumber=-2
  LAS_SLASpdLimitUnit_sat : Saturate  UpperLimit=0  LowerLimit=0
  LAS_SLASpdLimitUnit_st : Sum  Inputs=+-
  output1 : Outport
  output2 : Outport  Port=2
  output3 : Outport  Port=3
  output4 : Outport  Port=4
  output5 : Outport  Port=5
  output6 : Outport  Port=6
  output7 : Outport  Port=7
  output8 : Outport  Port=8
  wires:
  LAS_SLASpdLimitUnit/1 -> LAS_SLASpdLimitUnit_sat/1
  LAS_SLASpdLimitUnit_sat/1 -> LAS_SLASpdLimitUnit_st/1
  LAS_SLASpdLimitUnit_O/1 -> LAS_SLASpdLimitUnit_st/2
  LAS_SLASpdLimitUnit_st/1 -> LAS_SLASpdLimitUnit_D/1
  LAS_SLASpdLimitUnit_F/1 -> LAS_SLASpdLimitUnit_D/2
  LAS_SLASpdLimitUnit_D/1 -> LAS_SLASpdLimitUnitRon/1
  LAS_SLASpdLimitUnitRon/1 -> LAS_SLASpdLimitUnit_S/1
  LAS_SLASpdLimitUnit_S/1 -> LAS_SLASpdLimitUnit_1sat/1
  LAS_SLASpdLimitUnit_1sat/1 -> LAS_SLASpdLimitUnit_Convert1/1
  LAS_SLASpdLimitUnit_Convert1/1 -> LAS_SLASpdLimitUnit_L/1
  LAS_SLASpdLimitUnit_L/1 -> LAS_SLASpdLimitUnit_Convert/1
  LAS_SLASpdLimitUnit_Convert/1 -> output1/1
  Constant2/1 -> output2/1
  Constant3/1 -> output3/1
  Constant4/1 -> output4/1
  Constant5/1 -> output5/1
  Constant6/1 -> output6/1
  Constant7/1 -> output7/1
  Constant8/1 -> output8/1

== system VCU_CS75_12_16_Test/长安CS75底盘程序，20ms一次/Output/Subsystem/28D/LAS_28D/LAS_SLAState ==
  LAS_SLAState : Inport
  Constant{1..4,6..8} (7 alike) : Constant  Value=0  OutDataTypeStr=uint8
  LAS_SLAStateRon : Rounding  Operator=round
  LAS_SLAState_1sat : Saturate  UpperLimit=28  LowerLimit=0
  LAS_SLAState_Convert : DataTypeConversion  OutDataTypeStr=uint8
  LAS_SLAState_Convert1 : DataTypeConversion  OutDataTypeStr=uint32
  LAS_SLAState_D : Product  Inputs=*/
  LAS_SLAState_F : Constant  OutDataTypeStr=single
  LAS_SLAState_L : simulink/Logic and Bit Operations/Bitwise Operator  logicop=AND  UseBitMask=on  BitMask=28  BitMaskRealWorld=Stored Integer
  LAS_SLAState_O : Constant  Value=0  OutDataTypeStr=single
  LAS_SLAState_S : ArithShift  BitShiftNumber=-2
  LAS_SLAState_sat : Saturate  UpperLimit=0  LowerLimit=0
  LAS_SLAState_st : Sum  Inputs=+-
  output1 : Outport
  output2 : Outport  Port=2
  output3 : Outport  Port=3
  output4 : Outport  Port=4
  output5 : Outport  Port=5
  output6 : Outport  Port=6
  output7 : Outport  Port=7
  output8 : Outport  Port=8
  wires:
  LAS_SLAState/1 -> LAS_SLAState_sat/1
  LAS_SLAState_sat/1 -> LAS_SLAState_st/1
  LAS_SLAState_O/1 -> LAS_SLAState_st/2
  LAS_SLAState_st/1 -> LAS_SLAState_D/1
  LAS_SLAState_F/1 -> LAS_SLAState_D/2
  LAS_SLAState_D/1 -> LAS_SLAStateRon/1
  LAS_SLAStateRon/1 -> LAS_SLAState_S/1
  LAS_SLAState_S/1 -> LAS_SLAState_1sat/1
  LAS_SLAState_1sat/1 -> LAS_SLAState_Convert1/1
  LAS_SLAState_Convert1/1 -> LAS_SLAState_L/1
  LAS_SLAState_L/1 -> LAS_SLAState_Convert/1
  LAS_SLAState_Convert/1 -> output5/1
  Constant1/1 -> output1/1
  Constant2/1 -> output2/1
  Constant3/1 -> output3/1
  Constant4/1 -> output4/1
  Constant6/1 -> output6/1
  Constant7/1 -> output7/1
  Constant8/1 -> output8/1

== system VCU_CS75_12_16_Test/长安CS75底盘程序，20ms一次/Output/Subsystem/28D/LAS_28D/LAS_SteeringTorqueReq ==
  LAS_SteeringTorqueReq : Inport
  Constant{1..4,8} (5 alike) : Constant  Value=0  OutDataTypeStr=uint8
  LAS_SteeringTorqueReqBitCov : DataTypeConversion  OutDataTypeStr=uint32
  LAS_SteeringTorqueReqBitCov1 : DataTypeConversion  OutDataTypeStr=uint8
  LAS_SteeringTorqueReqCOV : DataTypeConversion  OutDataTypeStr=uint8
  LAS_SteeringTorqueReqCOV1 : DataTypeConversion  OutDataTypeStr=uint8
  LAS_SteeringTorqueReqRon : Rounding  Operator=round
  LAS_SteeringTorqueReq_1sat : Saturate  UpperLimit=262016  LowerLimit=0
  LAS_SteeringTorqueReq_And : simulink/Logic and Bit Operations/Bitwise Operator  logicop=AND  UseBitMask=off  NumInputPorts=2  BitMask=bin2dec('11011001')  BitMaskRealWorld=Stored Integer
  LAS_SteeringTorqueReq_And1 : simulink/Logic and Bit Operations/Bitwise Operator  logicop=AND  UseBitMask=off  NumInputPorts=2  BitMask=bin2dec('11011001')  BitMaskRealWorld=Stored Integer
  LAS_SteeringTorqueReq_And1_C : Constant  Value=255  OutDataTypeStr=uint32
  LAS_SteeringTorqueReq_And_C : Constant  Value=65535
  LAS_SteeringTorqueReq_Convert : DataTypeConversion  OutDataTypeStr=uint32
  LAS_SteeringTorqueReq_D : Product  Inputs=*/
  LAS_SteeringTorqueReq_D1 : Product  Inputs=*/
  LAS_SteeringTorqueReq_D2 : Product  Inputs=*/
  LAS_SteeringTorqueReq_F : Constant  Value=0.01  OutDataTypeStr=single
  LAS_SteeringTorqueReq_L : simulink/Logic and Bit Operations/Bitwise Operator  logicop=AND  UseBitMask=on  BitMask=262016  BitMaskRealWorld=Stored Integer
  LAS_SteeringTorqueReq_O : Constant  Value=-8  OutDataTypeStr=single
  LAS_SteeringTorqueReq_S : ArithShift  BitShiftNumber=-7
  LAS_SteeringTorqueReq_sat : Saturate  UpperLimit=12.47  LowerLimit=-8
  LAS_SteeringTorqueReq_st : Sum  Inputs=+-
  LAS_SteeringTorqueReqoutput5_C : Constant  Value=65536
  LAS_SteeringTorqueReqoutput6_C : Constant  Value=256
  output1 : Outport
  output2 : Outport  Port=2
  output3 : Outport  Port=3
  output4 : Outport  Port=4
  output5 : Outport  Port=5
  output6 : Outport  Port=6
  output7 : Outport  Port=7
  output8 : Outport  Port=8
  wires:
  LAS_SteeringTorqueReq/1 -> LAS_SteeringTorqueReq_sat/1
  LAS_SteeringTorqueReq_sat/1 -> LAS_SteeringTorqueReq_st/1
  LAS_SteeringTorqueReq_O/1 -> LAS_SteeringTorqueReq_st/2
  LAS_SteeringTorqueReq_st/1 -> LAS_SteeringTorqueReq_D/1
  LAS_SteeringTorqueReq_F/1 -> LAS_SteeringTorqueReq_D/2
  LAS_SteeringTorqueReq_D/1 -> LAS_SteeringTorqueReqRon/1
  LAS_SteeringTorqueReqRon/1 -> LAS_SteeringTorqueReq_S/1
  LAS_SteeringTorqueReq_S/1 -> LAS_SteeringTorqueReq_1sat/1
  LAS_SteeringTorqueReq_1sat/1 -> LAS_SteeringTorqueReq_Convert/1
  LAS_SteeringTorqueReq_Convert/1 -> LAS_SteeringTorqueReq_L/1
  LAS_SteeringTorqueReq_L/1 -> LAS_SteeringTorqueReq_D1/1, LAS_SteeringTorqueReq_And/1, LAS_SteeringTorqueReq_And1/1
  LAS_SteeringTorqueReqoutput5_C/1 -> LAS_SteeringTorqueReq_D1/2
  LAS_SteeringTorqueReq_D1/1 -> LAS_SteeringTorqueReqCOV/1
  LAS_SteeringTorqueReqCOV/1 -> output5/1
  LAS_SteeringTorqueReq_And_C/1 -> LAS_SteeringTorqueReqBitCov/1
  LAS_SteeringTorqueReqBitCov/1 -> LAS_SteeringTorqueReq_And/2
  LAS_SteeringTorqueReq_And/1 -> LAS_SteeringTorqueReq_D2/1
  LAS_SteeringTorqueReqoutput6_C/1 -> LAS_SteeringTorqueReq_D2/2
  LAS_SteeringTorqueReq_D2/1 -> LAS_SteeringTorqueReqCOV1/1
  LAS_SteeringTorqueReqCOV1/1 -> output6/1
  LAS_SteeringTorqueReq_And1_C/1 -> LAS_SteeringTorqueReq_And1/2
  LAS_SteeringTorqueReq_And1/1 -> LAS_SteeringTorqueReqBitCov1/1
  LAS_SteeringTorqueReqBitCov1/1 -> output7/1
  Constant1/1 -> output1/1
  Constant2/1 -> output2/1
  Constant3/1 -> output3/1
  Constant4/1 -> output4/1
  Constant8/1 -> output8/1

== system VCU_CS75_12_16_Test/长安CS75底盘程序，20ms一次/Output/Subsystem/28D/LAS_28D/LAS_TakeoverReq ==
  LAS_TakeoverReq : Inport
  Constant{1,3..8} (7 alike) : Constant  Value=0  OutDataTypeStr=uint8
  LAS_TakeoverReqRon : Rounding  Operator=round
  LAS_TakeoverReq_1sat : Saturate  UpperLimit=4  LowerLimit=0
  LAS_TakeoverReq_Convert : DataTypeConversion  OutDataTypeStr=uint8
  LAS_TakeoverReq_Convert1 : DataTypeConversion  OutDataTypeStr=uint32
  LAS_TakeoverReq_D : Product  Inputs=*/
  LAS_TakeoverReq_F : Constant  OutDataTypeStr=single
  LAS_TakeoverReq_L : simulink/Logic and Bit Operations/Bitwise Operator  logicop=AND  UseBitMask=on  BitMask=4  BitMaskRealWorld=Stored Integer
  LAS_TakeoverReq_O : Constant  Value=0  OutDataTypeStr=single
  LAS_TakeoverReq_S : ArithShift  BitShiftNumber=-2
  LAS_TakeoverReq_sat : Saturate  UpperLimit=1  LowerLimit=0
  LAS_TakeoverReq_st : Sum  Inputs=+-
  output1 : Outport
  output2 : Outport  Port=2
  output3 : Outport  Port=3
  output4 : Outport  Port=4
  output5 : Outport  Port=5
  output6 : Outport  Port=6
  output7 : Outport  Port=7
  output8 : Outport  Port=8
  wires:
  LAS_TakeoverReq/1 -> LAS_TakeoverReq_sat/1
  LAS_TakeoverReq_sat/1 -> LAS_TakeoverReq_st/1
  LAS_TakeoverReq_O/1 -> LAS_TakeoverReq_st/2
  LAS_TakeoverReq_st/1 -> LAS_TakeoverReq_D/1
  LAS_TakeoverReq_F/1 -> LAS_TakeoverReq_D/2
  LAS_TakeoverReq_D/1 -> LAS_TakeoverReqRon/1
  LAS_TakeoverReqRon/1 -> LAS_TakeoverReq_S/1
  LAS_TakeoverReq_S/1 -> LAS_TakeoverReq_1sat/1
  LAS_TakeoverReq_1sat/1 -> LAS_TakeoverReq_Convert1/1
  LAS_TakeoverReq_Convert1/1 -> LAS_TakeoverReq_L/1
  LAS_TakeoverReq_L/1 -> LAS_TakeoverReq_Convert/1
  LAS_TakeoverReq_Convert/1 -> output2/1
  Constant1/1 -> output1/1
  Constant3/1 -> output3/1
  Constant4/1 -> output4/1
  Constant5/1 -> output5/1
  Constant6/1 -> output6/1
  Constant7/1 -> output7/1
  Constant8/1 -> output8/1

== system VCU_CS75_12_16_Test/长安CS75底盘程序，20ms一次/Output/Subsystem/28D/LAS_28D/RollingConter ==
  RollingConter : Inport
  Constant{1..6,8} (7 alike) : Constant  Value=0  OutDataTypeStr=uint8
  RollingConterRon : Rounding  Operator=round
  RollingConter_1sat : Saturate  UpperLimit=15  LowerLimit=0
  RollingConter_Convert : DataTypeConversion  OutDataTypeStr=uint8
  RollingConter_Convert1 : DataTypeConversion  OutDataTypeStr=uint32
  RollingConter_D : Product  Inputs=*/
  RollingConter_F : Constant  OutDataTypeStr=single
  RollingConter_L : simulink/Logic and Bit Operations/Bitwise Operator  logicop=AND  UseBitMask=on  BitMask=15  BitMaskRealWorld=Stored Integer
  RollingConter_O : Constant  Value=0  OutDataTypeStr=single
  RollingConter_S : ArithShift
  RollingConter_sat : Saturate  UpperLimit=0  LowerLimit=0
  RollingConter_st : Sum  Inputs=+-
  output1 : Outport
  output2 : Outport  Port=2
  output3 : Outport  Port=3
  output4 : Outport  Port=4
  output5 : Outport  Port=5
  output6 : Outport  Port=6
  output7 : Outport  Port=7
  output8 : Outport  Port=8
  wires:
  RollingConter/1 -> RollingConter_sat/1
  RollingConter_sat/1 -> RollingConter_st/1
  RollingConter_O/1 -> RollingConter_st/2
  RollingConter_st/1 -> RollingConter_D/1
  RollingConter_F/1 -> RollingConter_D/2
  RollingConter_D/1 -> RollingConterRon/1
  RollingConterRon/1 -> RollingConter_S/1
  RollingConter_S/1 -> RollingConter_1sat/1
  RollingConter_1sat/1 -> RollingConter_Convert1/1
  RollingConter_Convert1/1 -> RollingConter_L/1
  RollingConter_L/1 -> RollingConter_Convert/1
  RollingConter_Convert/1 -> output7/1
  Constant1/1 -> output1/1
  Constant2/1 -> output2/1
  Constant3/1 -> output3/1
  Constant4/1 -> output4/1
  Constant5/1 -> output5/1
  Constant6/1 -> output6/1
  Constant8/1 -> output8/1

== system VCU_CS75_12_16_Test/长安CS75底盘程序，20ms一次/Output/Subsystem/2E4/ACC_2E4/ACC_ACCTargetAcceleration ==
  ACC_ACCTargetAcceleration : Inport
  ACC_ACCTargetAccelerationRon : Rounding  Operator=round
  ACC_ACCTargetAcceleration_1sat : Saturate  UpperLimit=255  LowerLimit=0
  ACC_ACCTargetAcceleration_Convert : DataTypeConversion  OutDataTypeStr=uint8
  ACC_ACCTargetAcceleration_Convert1 : DataTypeConversion  OutDataTypeStr=uint32
  ACC_ACCTargetAcceleration_D : Product  Inputs=*/
  ACC_ACCTargetAcceleration_F : Constant  Value=0.05  OutDataTypeStr=single
  ACC_ACCTargetAcceleration_L : simulink/Logic and Bit Operations/Bitwise Operator  logicop=AND  UseBitMask=on  BitMask=255  BitMaskRealWorld=Stored Integer
  ACC_ACCTargetAcceleration_O : Constant  Value=-5  OutDataTypeStr=single
  ACC_ACCTargetAcceleration_S : ArithShift
  ACC_ACCTargetAcceleration_sat : Saturate  UpperLimit=7.75  LowerLimit=-5
  ACC_ACCTargetAcceleration_st : Sum  Inputs=+-
  Constant{1,3..8} (7 alike) : Constant  Value=0  OutDataTypeStr=uint8
  output1 : Outport
  output2 : Outport  Port=2
  output3 : Outport  Port=3
  output4 : Outport  Port=4
  output5 : Outport  Port=5
  output6 : Outport  Port=6
  output7 : Outport  Port=7
  output8 : Outport  Port=8
  wires:
  ACC_ACCTargetAcceleration/1 -> ACC_ACCTargetAcceleration_sat/1
  ACC_ACCTargetAcceleration_sat/1 -> ACC_ACCTargetAcceleration_st/1
  ACC_ACCTargetAcceleration_O/1 -> ACC_ACCTargetAcceleration_st/2
  ACC_ACCTargetAcceleration_st/1 -> ACC_ACCTargetAcceleration_D/1
  ACC_ACCTargetAcceleration_F/1 -> ACC_ACCTargetAcceleration_D/2
  ACC_ACCTargetAcceleration_D/1 -> ACC_ACCTargetAccelerationRon/1
  ACC_ACCTargetAccelerationRon/1 -> ACC_ACCTargetAcceleration_S/1
  ACC_ACCTargetAcceleration_S/1 -> ACC_ACCTargetAcceleration_1sat/1
  ACC_ACCTargetAcceleration_1sat/1 -> ACC_ACCTargetAcceleration_Convert1/1
  ACC_ACCTargetAcceleration_Convert1/1 -> ACC_ACCTargetAcceleration_L/1
  ACC_ACCTargetAcceleration_L/1 -> ACC_ACCTargetAcceleration_Convert/1
  ACC_ACCTargetAcceleration_Convert/1 -> output2/1
  Constant1/1 -> output1/1
  Constant3/1 -> output3/1
  Constant4/1 -> output4/1
  Constant5/1 -> output5/1
  Constant6/1 -> output6/1
  Constant7/1 -> output7/1
  Constant8/1 -> output8/1

== system VCU_CS75_12_16_Test/长安CS75底盘程序，20ms一次/Output/Subsystem/2E4/ACC_2E4/ACC_CDDAxEnable ==
  ACC_CDDAxEnable : Inport
  ACC_CDDAxEnableRon : Rounding  Operator=round
  ACC_CDDAxEnable_1sat : Saturate  UpperLimit=1  LowerLimit=0
  ACC_CDDAxEnable_Convert : DataTypeConversion  OutDataTypeStr=uint8
  ACC_CDDAxEnable_Convert1 : DataTypeConversion  OutDataTypeStr=uint32
  ACC_CDDAxEnable_D : Product  Inputs=*/
  ACC_CDDAxEnable_F : Constant  OutDataTypeStr=single
  ACC_CDDAxEnable_L : simulink/Logic and Bit Operations/Bitwise Operator  logicop=AND  UseBitMask=on  BitMask=1  BitMaskRealWorld=Stored Integer
  ACC_CDDAxEnable_O : Constant  Value=0  OutDataTypeStr=single
  ACC_CDDAxEnable_S : ArithShift
  ACC_CDDAxEnable_sat : Saturate  UpperLimit=1  LowerLimit=0
  ACC_CDDAxEnable_st : Sum  Inputs=+-
  Constant{2..8} (7 alike) : Constant  Value=0  OutDataTypeStr=uint8
  output1 : Outport
  output2 : Outport  Port=2
  output3 : Outport  Port=3
  output4 : Outport  Port=4
  output5 : Outport  Port=5
  output6 : Outport  Port=6
  output7 : Outport  Port=7
  output8 : Outport  Port=8
  wires:
  ACC_CDDAxEnable/1 -> ACC_CDDAxEnable_sat/1
  ACC_CDDAxEnable_sat/1 -> ACC_CDDAxEnable_st/1
  ACC_CDDAxEnable_O/1 -> ACC_CDDAxEnable_st/2
  ACC_CDDAxEnable_st/1 -> ACC_CDDAxEnable_D/1
  ACC_CDDAxEnable_F/1 -> ACC_CDDAxEnable_D/2
  ACC_CDDAxEnable_D/1 -> ACC_CDDAxEnableRon/1
  ACC_CDDAxEnableRon/1 -> ACC_CDDAxEnable_S/1
  ACC_CDDAxEnable_S/1 -> ACC_CDDAxEnable_1sat/1
  ACC_CDDAxEnable_1sat/1 -> ACC_CDDAxEnable_Convert1/1
  ACC_CDDAxEnable_Convert1/1 -> ACC_CDDAxEnable_L/1
  ACC_CDDAxEnable_L/1 -> ACC_CDDAxEnable_Convert/1
  ACC_CDDAxEnable_Convert/1 -> output1/1
  Constant2/1 -> output2/1
  Constant3/1 -> output3/1
  Constant4/1 -> output4/1
  Constant5/1 -> output5/1
  Constant6/1 -> output6/1
  Constant7/1 -> output7/1
  Constant8/1 -> output8/1

== system VCU_CS75_12_16_Test/长安CS75底盘程序，20ms一次/Output/Subsystem/2E4/ACC_2E4/ACC_CheckSum_id ==
  ACC_CheckSum_id : Inport
  ACC_CheckSum_idRon : Rounding  Operator=round
  ACC_CheckSum_id_1sat : Saturate  UpperLimit=255  LowerLimit=0
  ACC_CheckSum_id_Convert : DataTypeConversion  OutDataTypeStr=uint8
  ACC_CheckSum_id_Convert1 : DataTypeConversion  OutDataTypeStr=uint32
  ACC_CheckSum_id_D : Product  Inputs=*/
  ACC_CheckSum_id_F : Constant  OutDataTypeStr=single
  ACC_CheckSum_id_L : simulink/Logic and Bit Operations/Bitwise Operator  logicop=AND  UseBitMask=on  BitMask=255  BitMaskRealWorld=Stored Integer
  ACC_CheckSum_id_O : Constant  Value=0  OutDataTypeStr=single
  ACC_CheckSum_id_S : ArithShift
  ACC_CheckSum_id_sat : Saturate  UpperLimit=255  LowerLimit=0
  ACC_CheckSum_id_st : Sum  Inputs=+-
  Constant{1..7} (7 alike) : Constant  Value=0  OutDataTypeStr=uint8
  output1 : Outport
  output2 : Outport  Port=2
  output3 : Outport  Port=3
  output4 : Outport  Port=4
  output5 : Outport  Port=5
  output6 : Outport  Port=6
  output7 : Outport  Port=7
  output8 : Outport  Port=8
  wires:
  ACC_CheckSum_id/1 -> ACC_CheckSum_id_sat/1
  ACC_CheckSum_id_sat/1 -> ACC_CheckSum_id_st/1
  ACC_CheckSum_id_O/1 -> ACC_CheckSum_id_st/2
  ACC_CheckSum_id_st/1 -> ACC_CheckSum_id_D/1
  ACC_CheckSum_id_F/1 -> ACC_CheckSum_id_D/2
  ACC_CheckSum_id_D/1 -> ACC_CheckSum_idRon/1
  ACC_CheckSum_idRon/1 -> ACC_CheckSum_id_S/1
  ACC_CheckSum_id_S/1 -> ACC_CheckSum_id_1sat/1
  ACC_CheckSum_id_1sat/1 -> ACC_CheckSum_id_Convert1/1
  ACC_CheckSum_id_Convert1/1 -> ACC_CheckSum_id_L/1
  ACC_CheckSum_id_L/1 -> ACC_CheckSum_id_Convert/1
  ACC_CheckSum_id_Convert/1 -> output8/1
  Constant1/1 -> output1/1
  Constant2/1 -> output2/1
  Constant3/1 -> output3/1
  Constant4/1 -> output4/1
  Constant5/1 -> output5/1
  Constant6/1 -> output6/1
  Constant7/1 -> output7/1

== system VCU_CS75_12_16_Test/长安CS75底盘程序，20ms一次/Output/Subsystem/2E4/ACC_2E4/ACC_DecToStop ==
  ACC_DecToStop : Inport
  ACC_DecToStopRon : Rounding  Operator=round
  ACC_DecToStop_1sat : Saturate  UpperLimit=2  LowerLimit=0
  ACC_DecToStop_Convert : DataTypeConversion  OutDataTypeStr=uint8
  ACC_DecToStop_Convert1 : DataTypeConversion  OutDataTypeStr=uint32
  ACC_DecToStop_D : Product  Inputs=*/
  ACC_DecToStop_F : Constant  OutDataTypeStr=single
  ACC_DecToStop_L : simulink/Logic and Bit Operations/Bitwise Operator  logicop=AND  UseBitMask=on  BitMask=2  BitMaskRealWorld=Stored Integer
  ACC_DecToStop_O : Constant  Value=0  OutDataTypeStr=single
  ACC_DecToStop_S : ArithShift  BitShiftNumber=-1
  ACC_DecToStop_sat : Saturate  UpperLimit=1  LowerLimit=0
  ACC_DecToStop_st : Sum  Inputs=+-
  Constant{2..8} (7 alike) : Constant  Value=0  OutDataTypeStr=uint8
  output1 : Outport
  output2 : Outport  Port=2
  output3 : Outport  Port=3
  output4 : Outport  Port=4
  output5 : Outport  Port=5
  output6 : Outport  Port=6
  output7 : Outport  Port=7
  output8 : Outport  Port=8
  wires:
  ACC_DecToStop/1 -> ACC_DecToStop_sat/1
  ACC_DecToStop_sat/1 -> ACC_DecToStop_st/1
  ACC_DecToStop_O/1 -> ACC_DecToStop_st/2
  ACC_DecToStop_st/1 -> ACC_DecToStop_D/1
  ACC_DecToStop_F/1 -> ACC_DecToStop_D/2
  ACC_DecToStop_D/1 -> ACC_DecToStopRon/1
  ACC_DecToStopRon/1 -> ACC_DecToStop_S/1
  ACC_DecToStop_S/1 -> ACC_DecToStop_1sat/1
  ACC_DecToStop_1sat/1 -> ACC_DecToStop_Convert1/1
  ACC_DecToStop_Convert1/1 -> ACC_DecToStop_L/1
  ACC_DecToStop_L/1 -> ACC_DecToStop_Convert/1
  ACC_DecToStop_Convert/1 -> output1/1
  Constant2/1 -> output2/1
  Constant3/1 -> output3/1
  Constant4/1 -> output4/1
  Constant5/1 -> output5/1
  Constant6/1 -> output6/1
  Constant7/1 -> output7/1
  Constant8/1 -> output8/1
